simulink model "linear_Convolution"  (R2021a)
settings: Solver=VariableStepAuto  StartTime=0.0  StopTime=10.0  RelTol=1e-3
libraries: dspsigops x1, dspsrcs4 x1
settings Model: Creator=hythe  LastModifiedBy=BluRay
settings SolverCC: AlgebraicLoopSolver=TrustRegion
settings DebuggingCC: SFMachineParentedDataDiag=warning

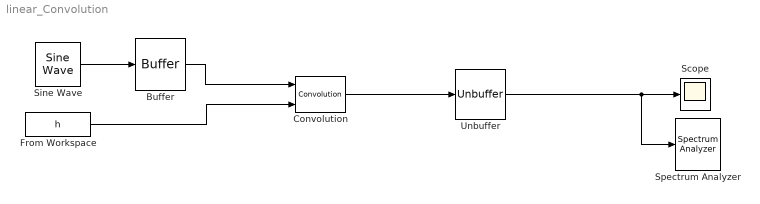
== system linear_Convolution ==
  Buffer : Buffer  N=8000  OutputFrames=off
  Convolution : dspsigops/Convolution  domain=Time  roundingMode=Floor  overflowMode=off  outputDataTypeStr=Inherit: Same as accumulator  outputMin=[]  outputMax=[]  outputLastDataTypeStr=Inherit: Same as accumulator
      settings: SourceProductBaseCode=DS
  From Workspace : FromWorkspace  VariableName=h  SampleTime=1
  Scope : Scope
  Sine Wave : dspsrcs4/Sine Wave  Amplitude=1  Frequency=100  Phase=0  SampleMode=Discrete  OutComplex=Real  CompMethod=Trigonometric fcn  TableSize=Speed  SampleTime=1/8000  SamplesPerFrame=1  ResetState=Restart at time zero  OutputFrames=off  dataType=double  wordLen=16  udDataType=sfix(16)  fracBitsMode=Best precision  numFracBits=15  OutDataTypeStr=double  LastOutDataTypeStr=double
  Spectrum Analyzer : SpectrumAnalyzer
  Unbuffer : Unbuffer
  wires:
  Sine Wave/1 -> Buffer/1
  Unbuffer/1 -> Spectrum Analyzer/1, Scope/1
  Buffer/1 -> Convolution/1
  From Workspace/1 -> Convolution/2
  Convolution/1 -> Unbuffer/1
